simulink model "BolandLab4"  (R2024a)
settings: Solver=ode5  StartTime=0.0  StopTime=1000  RelTol=1e-3
settings Model: Creator=Test  LastModifiedBy=Test

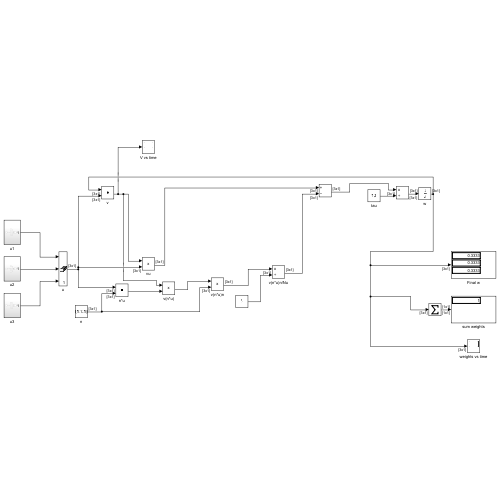
[thumbnail: Simulink's stored preview of the top-level diagram]
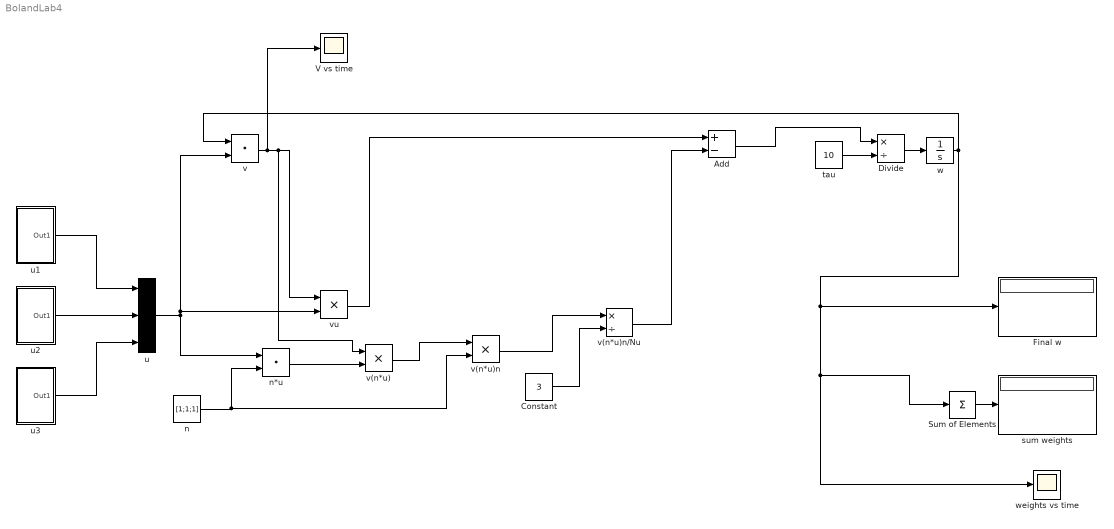
== system BolandLab4 ==
  Add : Sum  Inputs=+-
  Constant : Constant  Value=3
  Divide : Product  Inputs=*/
  Final w : Display
  Sum of Elements : Sum  Inputs=+
  V vs time : Scope
  n : Constant  Value=[1;1;1]  VectorParams1D=off
  n*u : DotProduct  OutDataTypeStr=Inherit: Inherit via internal rule
  sum weights : Display
  tau : Constant  Value=10
  u : Concatenate  NumInputs=3  Mode=Multidimensional array
  u1 : Subsystem
  u2 : Subsystem
  u3 : Subsystem
  v : DotProduct  OutDataTypeStr=Inherit: Inherit via internal rule
  v(n*u) : Product
  v(n*u)n : Product
  v(n*u)n/Nu : Product  Inputs=*/
  vu : Product
  w : Integrator  InitialCondition=[1/3;1/3;1/3]
  weights vs time : Scope
  wires:
  u2/1(Out1) -> u/2
  u1/1(Out1) -> u/1
  u3/1(Out1) -> u/3
  u/1 -> vu/2, v/2, n*u/1
  v/1 -> V vs time/1, vu/1, v(n*u)/1
  Divide/1 -> w/1
  tau/1 -> Divide/2
  Add/1 -> Divide/1
  vu/1 -> Add/1
  n/1 -> v(n*u)n/2, n*u/2
  n*u/1 -> v(n*u)/2
  v(n*u)/1 -> v(n*u)n/1
  v(n*u)n/1 -> v(n*u)n/Nu/1
  Constant/1 -> v(n*u)n/Nu/2
  v(n*u)n/Nu/1 -> Add/2
  w/1 -> v/1, Sum of Elements/1, weights vs time/1, Final w/1
  Sum of Elements/1 -> sum weights/1

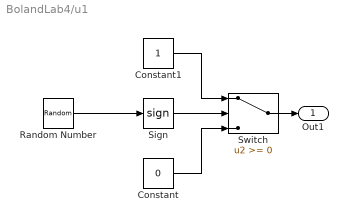
== system BolandLab4/u1 ==
  Constant : Constant  Value=0
  Constant1 : Constant
  Random Number : RandomNumber  Mean=0.1  Seed=3  SampleTime=1
  Sign : Signum
  Switch : Switch  SaturateOnIntegerOverflow=off  InputSameDT=off
  Out1 : Outport
  wires:
  Sign/1 -> Switch/2
  Random Number/1 -> Sign/1
  Constant/1 -> Switch/3
  Constant1/1 -> Switch/1
  Switch/1 -> Out1/1

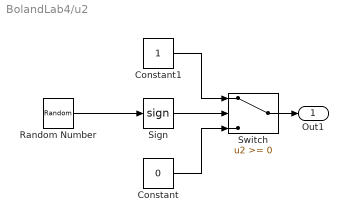
== system BolandLab4/u2 ==
  Constant : Constant  Value=0
  Constant1 : Constant
  Random Number : RandomNumber  Seed=3  SampleTime=1
  Sign : Signum
  Switch : Switch  SaturateOnIntegerOverflow=off  InputSameDT=off
  Out1 : Outport
  wires:
  Sign/1 -> Switch/2
  Random Number/1 -> Sign/1
  Constant/1 -> Switch/3
  Constant1/1 -> Switch/1
  Switch/1 -> Out1/1

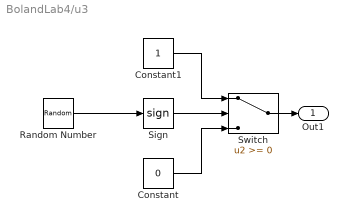
== system BolandLab4/u3 ==
  Constant : Constant  Value=0
  Constant1 : Constant
  Random Number : RandomNumber  Seed=3  SampleTime=1
  Sign : Signum
  Switch : Switch  SaturateOnIntegerOverflow=off  InputSameDT=off
  Out1 : Outport
  wires:
  Sign/1 -> Switch/2
  Random Number/1 -> Sign/1
  Constant/1 -> Switch/3
  Constant1/1 -> Switch/1
  Switch/1 -> Out1/1
